simulink model "Q2"  (R2022b)
settings: Solver=VariableStepAuto  StartTime=0.0  StopTime=10.0  RelTol=1e-3
undefined symbols (not defined in the file or in its folder): A_dynamic_matrix, B_dynamic_matrix, v
settings Model: Creator=Miakho  LastModifiedBy=Miakho

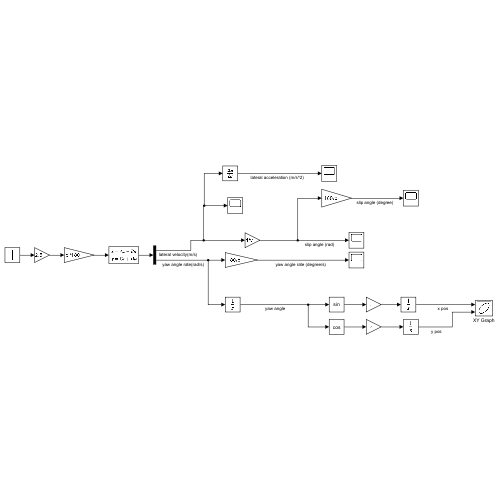
[thumbnail: Simulink's stored preview of the top-level diagram]
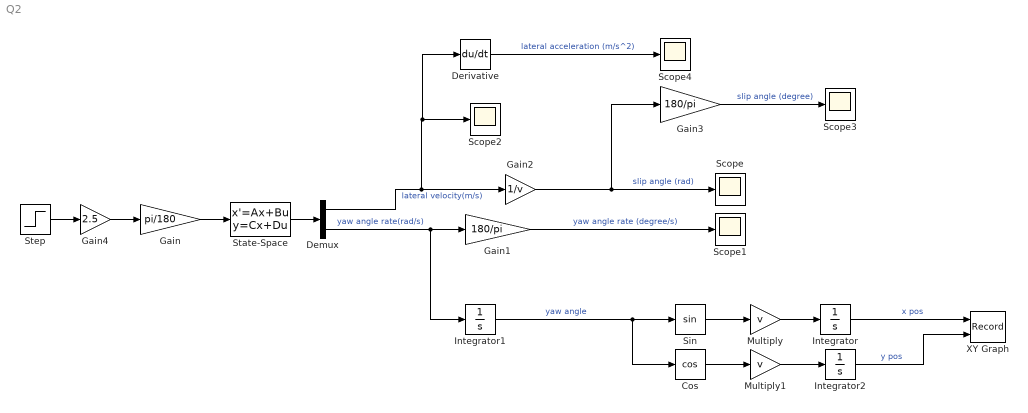
== system Q2 ==
  Cos : Trigonometry  Operator=cos
  Demux : Demux  Outputs=2
  Derivative : Derivative
  Gain : Gain  Gain=pi/180
  Gain1 : Gain  Gain=180/pi
  Gain2 : Gain  Gain=1/v
  Gain3 : Gain  Gain=180/pi
  Gain4 : Gain  Gain=2.5
  Integrator : Integrator
  Integrator1 : Integrator
  Integrator2 : Integrator
  Multiply : Gain  Gain=v
  Multiply1 : Gain  Gain=v
  Scope{,1..4} (5 alike) : Scope
  Sin : Trigonometry
  State-Space : StateSpace  A=A_dynamic_matrix  B=B_dynamic_matrix  C=[1 0; 0 1]  D=[0; 0]  InitialCondition=0
  Step : Step  Time=5  SampleTime=0
  XY Graph : Record  FileSettingsInternal="{\"entries\":[{\"content\":{\"excelSettings\":{\"content\":{},\"type\":\"Streamout.ExcelSettings\"}},\"type\":\"Streamout.FileSettingStorage\",\"uuid\":\"e2a7757d-8c5e-4edd-ae76-481941e8754d\"}],\"packageUris\":[\"http://schema.mathworks.com/mf0/streamout_blocks/R2020a\"],\"version\":\"1.0\"}"  Layout=[1 1]  SignalsInternal="{\"entries\":[{\"content\":{\"signals\":[{\"content\":{\"blockPath\":[\"Q2/XY Graph\"],\"channel\":[],\"dimensions\":[1],\"domain\":\"Q2/XY Graph\",\"lineColor\":\"#a2142f\",\"plots\":[1],\"port\":1,\"sid\":[\"\"],\"signalID\":164,\"signalName\":\"x pos\"},\"type\":\"RecordBlkView.Signal\",\"uuid\":\"b75b6a1b-2e45-4181-b7c2-bb769bfad797\"},{\"content\":{\"blockPath\":[\"Q2/XY Graph\"],\"channel\":[],\"dimensions\":[1],\"domain\":\"Q2/XY Graph\",\"lineColor\":\"#139fff\",\"plots\":[1],\"port\":2,\"sid\":[\"\"],\"signalID\":168,\"signalName\":\"y pos\"},\"type\":\"RecordBlkView.Signal\",\"uuid\":\"f0118be3-9fc1-4042-8aab-26789f39c3df\"}]},\"type\":\"RecordBlkView.InputSignals\",\"uuid\":\"30ce369e-b103-459b-926b-cf3152b4d80c\"}],\"packageUris\":[\"http://schema.mathworks.com/mf0/streamout_blocks/R2020a\"],\"version\":\"1.0\"}"  VisualizationBindings="{\"xyplotplugin\":{\"info\":[{\"series\":[{\"bindingParametersList\":[{\"parameter\":\"X-Axis\",\"signalID\":164,\"signalName\":\"x pos\"},{\"parameter\":\"Y-Axis\",\"signalID\":168,\"signalName\":\"y pos\"}],\"seriesID\":20040}],\"subplotID\":1}]}}"  CompatibilityTag=XY
  wires:
  Gain4/1 -> Gain/1
  State-Space/1 -> Demux/1
  Demux/1 -> Gain2/1, Derivative/1, Scope2/1  "lateral velocity(m/s)"
  Demux/2 -> Integrator1/1, Gain1/1  "yaw angle rate(rad/s)"
  Gain/1 -> State-Space/1
  Gain1/1 -> Scope1/1  "yaw angle rate (degree/s)"
  Gain2/1 -> Gain3/1, Scope/1  "slip angle (rad)"
  Gain3/1 -> Scope3/1  "slip angle (degree)"
  Step/1 -> Gain4/1
  Derivative/1 -> Scope4/1  "lateral acceleration (m/s^2)"
  Integrator1/1 -> Cos/1, Sin/1  "yaw angle"
  Sin/1 -> Multiply/1
  Cos/1 -> Multiply1/1
  Multiply/1 -> Integrator/1
  Multiply1/1 -> Integrator2/1
  Integrator/1 -> XY Graph/1  "x pos"
  Integrator2/1 -> XY Graph/2  "y pos"
